simulink model "odasaki"  (R2022b)
settings: Solver=VariableStepAuto  StartTime=0.0  StopTime=inf  RelTol=1e-3
undefined symbols (not defined in the file or in its folder): Angular, Linear
libraries: robotlib x5
settings Model: Creator=oda  LastModifiedBy=oda

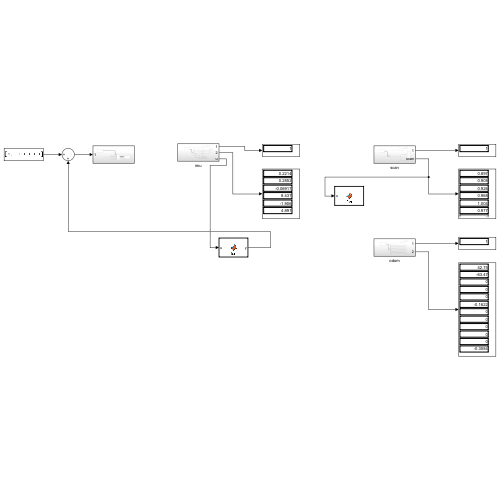
[thumbnail: Simulink's stored preview of the top-level diagram]
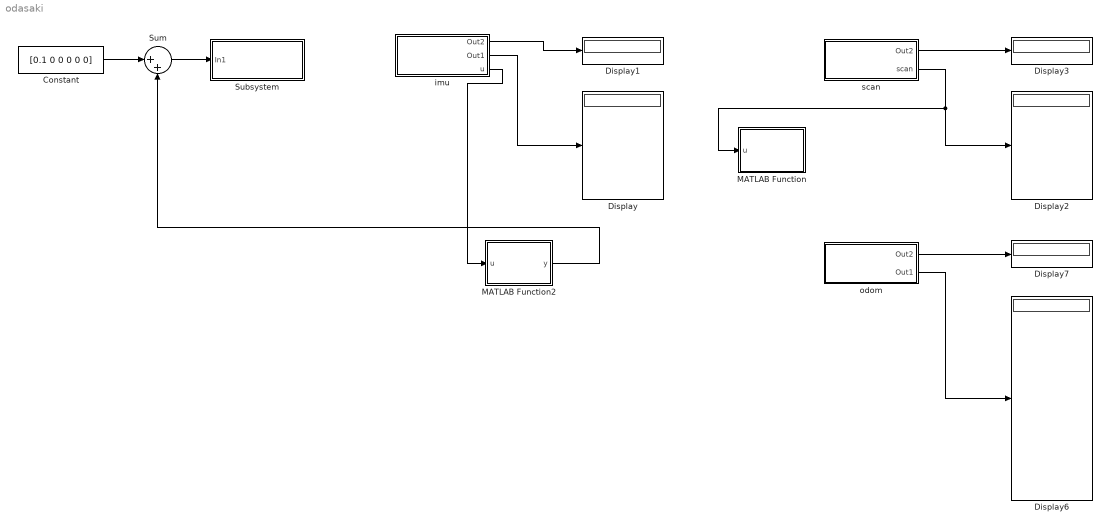
== system odasaki ==
  Constant : Constant  Value=[0.1 0 0 0 0 0]
  Display{,1..3,6..7} (6 alike) : Display
  MATLAB Function : MATLAB Function  TreatAsAtomicUnit=on
  MATLAB Function2 : MATLAB Function  TreatAsAtomicUnit=on
  Subsystem : Subsystem
  Sum : Sum  Inputs=|++
  imu : Subsystem
  odom : Subsystem
  scan : Subsystem
  wires:
  imu/2(Out1) -> Display/1
  imu/1(Out2) -> Display1/1
  scan/2(scan) -> MATLAB Function/1(u), Display2/1
  scan/1(Out2) -> Display3/1
  odom/1(Out2) -> Display7/1
  odom/2(Out1) -> Display6/1
  Constant/1 -> Sum/1
  Sum/1 -> Subsystem/1(In1)
  imu/3(u) -> MATLAB Function2/1(u)
  MATLAB Function2/1(y) -> Sum/2

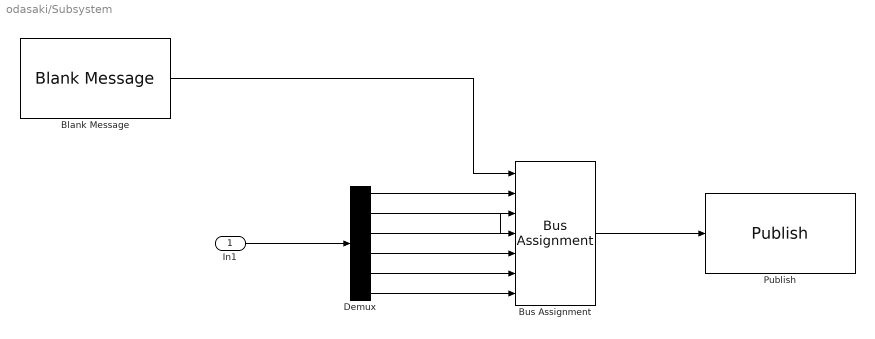
== system odasaki/Subsystem ==
  In1 : Inport
  Blank Message : robotlib/Blank Message  messageClass=Message  entityType=geometry_msgs/Twist  messageType=geometry_msgs/Twist  SampleTime=inf  legacyBusStruct=off
      settings: LibrarySourceBlock=roslib/ROS/Blank Message
  Bus Assignment : BusAssignment  AssignedSignals=Linear.X,Linear.Y,Linear.Z,Angular.X,Angular.Y,Angular.Z
  Demux : Demux  Outputs=6
  Publish : robotlib/Publish  topicSource=Specify your own  topic=/cmd_vel  messageType=geometry_msgs/Twist  legacyBusStruct=off  messageQueueLength=1
      settings: LibrarySourceBlock=roslib/ROS/Publish
  wires:
  In1/1 -> Demux/1
  Demux/1 -> Bus Assignment/2
  Bus Assignment/1 -> Publish/1
  Blank Message/1 -> Bus Assignment/1
  Demux/2 -> Bus Assignment/4
  Demux/3 -> Bus Assignment/3
  Demux/4 -> Bus Assignment/5
  Demux/5 -> Bus Assignment/6
  Demux/6 -> Bus Assignment/7

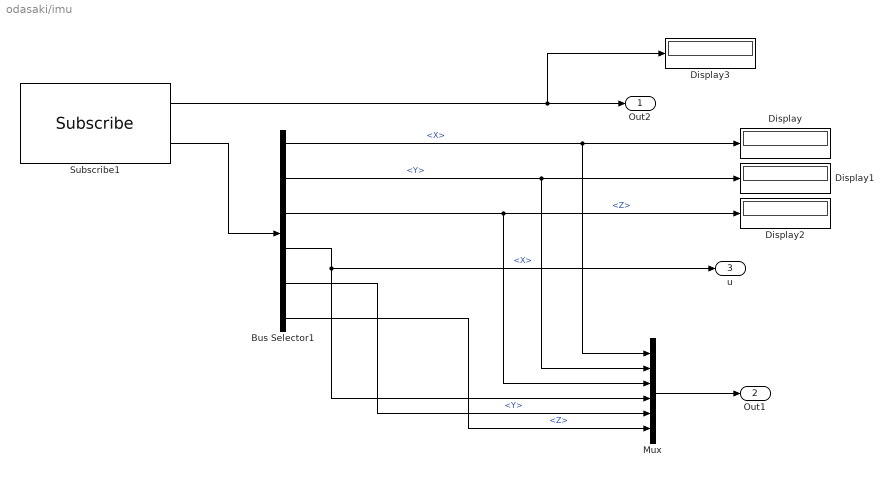
== system odasaki/imu ==
  Bus Selector1 : BusSelector  OutputSignals=AngularVelocity.X,AngularVelocity.Y,AngularVelocity.Z,LinearAcceleration.X,LinearAcceleration.Y,LinearAcceleration.Z
  Display{,1..3} (4 alike) : Display
  Mux : Mux  Inputs=6
  Subscribe1 : robotlib/Subscribe  topicSource=Specify your own  topic=/imu  messageType=sensor_msgs/Imu  SampleTime=0.1  legacyBusStruct=off  messageQueueLength=1
      settings: LibrarySourceBlock=roslib/ROS/Subscribe
  Out2 : Outport
  Out1 : Outport  Port=2
  u : Outport  Port=3
  wires:
  Mux/1 -> Out1/1
  Subscribe1/1 -> Display3/1, Out2/1
  Bus Selector1/1 -> Display/1, Mux/1  "<X>"
  Subscribe1/2 -> Bus Selector1/1
  Bus Selector1/2 -> Display1/1, Mux/2  "<Y>"
  Bus Selector1/3 -> Display2/1, Mux/3  "<Z>"
  Bus Selector1/6 -> Mux/6  "<Z>"
  Bus Selector1/5 -> Mux/5  "<Y>"
  Bus Selector1/4 -> u/1, Mux/4  "<X>"

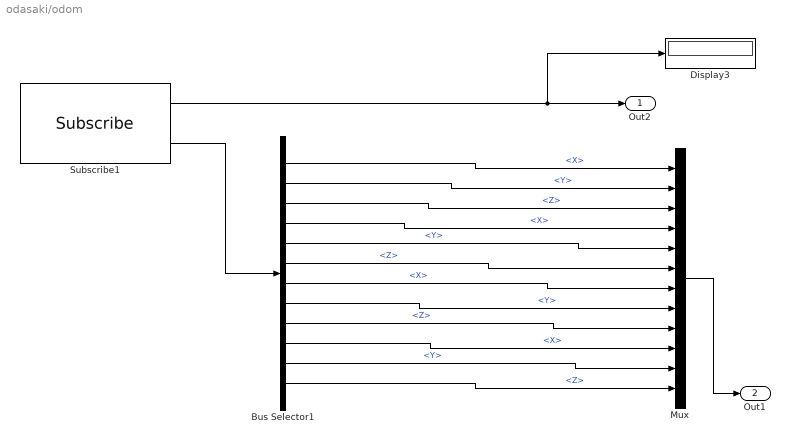
== system odasaki/odom ==
  Bus Selector1 : BusSelector  OutputSignals=Pose.Pose.Position.X,Pose.Pose.Position.Y,Pose.Pose.Position.Z,Pose.Pose.Orientation.X,Pose.Pose.Orientation.Y,Pose.Pose.Orientation.Z,Twist.Twist.Linear.X,Twist.Twist.Linear.Y,Twist.Twist.Linear.Z,Twist.Twist.Angular.X,Twist.Twist.Angular.Y,Twist.Twist.Angular.Z
  Display3 : Display
  Mux : Mux  Inputs=12
  Subscribe1 : robotlib/Subscribe  topicSource=Specify your own  topic=/odom  messageType=nav_msgs/Odometry  SampleTime=0.1  legacyBusStruct=off  messageQueueLength=1
      settings: LibrarySourceBlock=roslib/ROS/Subscribe
  Out2 : Outport
  Out1 : Outport  Port=2
  wires:
  Mux/1 -> Out1/1
  Subscribe1/1 -> Display3/1, Out2/1
  Bus Selector1/1 -> Mux/1  "<X>"
  Subscribe1/2 -> Bus Selector1/1
  Bus Selector1/2 -> Mux/2  "<Y>"
  Bus Selector1/3 -> Mux/3  "<Z>"
  Bus Selector1/4 -> Mux/4  "<X>"
  Bus Selector1/5 -> Mux/5  "<Y>"
  Bus Selector1/12 -> Mux/12  "<Z>"
  Bus Selector1/11 -> Mux/11  "<Y>"
  Bus Selector1/10 -> Mux/10  "<X>"
  Bus Selector1/9 -> Mux/9  "<Z>"
  Bus Selector1/8 -> Mux/8  "<Y>"
  Bus Selector1/7 -> Mux/7  "<X>"
  Bus Selector1/6 -> Mux/6  "<Z>"

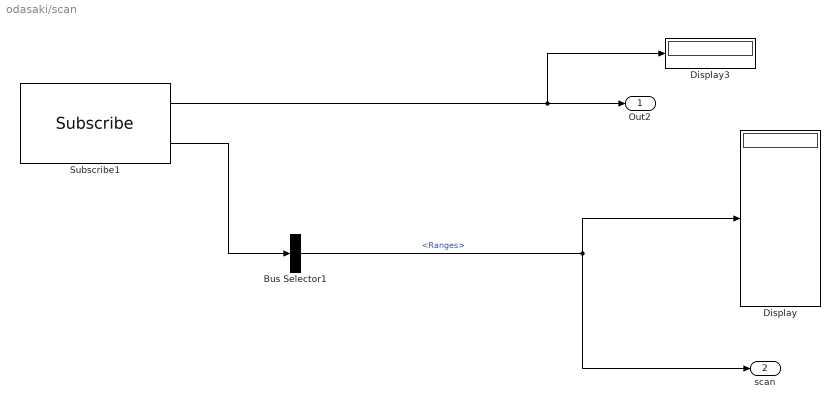
== system odasaki/scan ==
  Bus Selector1 : BusSelector  OutputSignals=Ranges
  Display : Display
  Display3 : Display
  Subscribe1 : robotlib/Subscribe  topicSource=Specify your own  topic=/scan  messageType=sensor_msgs/LaserScan  SampleTime=0.1  legacyBusStruct=off  messageQueueLength=1
      settings: LibrarySourceBlock=roslib/ROS/Subscribe
  Out2 : Outport
  scan : Outport  Port=2
  wires:
  Subscribe1/1 -> Display3/1, Out2/1
  Bus Selector1/1 -> scan/1, Display/1  "<Ranges>"
  Subscribe1/2 -> Bus Selector1/1

== matlab function odasaki/MATLAB Function2 ==
  data: u input; y output
function y = fcn(u)

if(u > 5)
    n = [-0.08 0 0 0 0 0];
elseif(u < -5)
    n = [0.08 0 0 0 0 0];
else
    n = [0 0 0 0 0 0];
end

y = n;

== matlab function odasaki/MATLAB Function ==
  data: u input
function fcn(u)
figure(1)
plot(u)
%y = u;
